simulink model "Bands2"  (R2018a)
settings: Solver=VariableStepAuto  StartTime=0.0  StopTime=0.001  RelTol=1e-3
undefined symbols (not defined in the file): fdesignblkfcn, G1, G2, gcbh, get, T
libraries: dspsrcs4 x1, dspxfrm3 x1, dspobslib x1
settings Model: Creator=Daniel  LastModifiedBy=Daniel

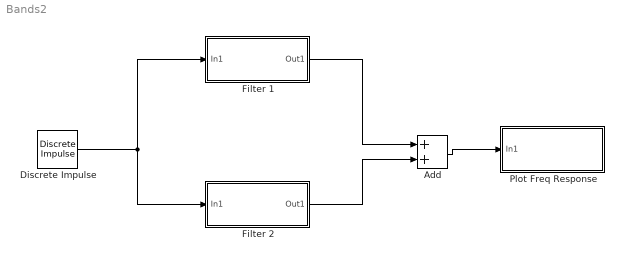
== system Bands2 ==
  Add : Sum
  Discrete Impulse : dspsrcs4/Discrete  Impulse  Delay=0  SampleTime=T  FrameSample=128  OutputFrames=off  dataType=double  isSigned=on  wordLen=16  udDataType=sfix(16)  fracBitsMode=Best precision  numFracBits=15  OutDataTypeStr=double  LastOutDataTypeStr=double
  Filter 1 : Subsystem
  Filter 2 : Subsystem
  Plot Freq Response : Subsystem
  wires:
  Discrete Impulse/1 -> Filter 2/1(In1), Filter 1/1(In1)
  Add/1 -> Plot Freq Response/1(In1)
  Filter 1/1(Out1) -> Add/1
  Filter 2/1(Out1) -> Add/2

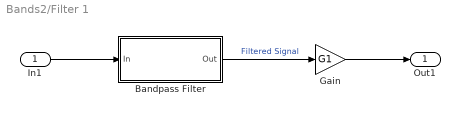
== system Bands2/Filter 1 ==
  In1 : Inport
  Bandpass Filter : Subsystem  DialogController=fdesignblkfcn  InitFcn=fdesignblkfcn(gcbh, {'InitFcn'});  mask(Bandpass Filter){}
      mask help: Design a bandpass filter
      settings: CopyFcn=fdesignblkfcn(gcbh, {'CopyFcn'});
      mask Help: helpview(mapfilelocation('dsp'), 'dspbandpassfilter');
      mask Display: disp('Bandpass');
  Gain : Gain  Gain=G1
  Out1 : Outport
  wires:
  Bandpass Filter/1(Out) -> Gain/1  "Filtered Signal"
  In1/1 -> Bandpass Filter/1(In)
  Gain/1 -> Out1/1

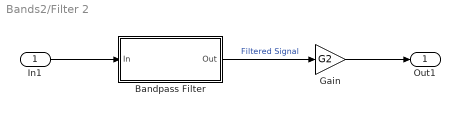
== system Bands2/Filter 2 ==
  In1 : Inport
  Bandpass Filter : Subsystem  DialogController=fdesignblkfcn  InitFcn=fdesignblkfcn(gcbh, {'InitFcn'});  mask(Bandpass Filter){}
      mask help: Design a bandpass filter
      settings: CopyFcn=fdesignblkfcn(gcbh, {'CopyFcn'});
      mask Help: helpview(mapfilelocation('dsp'), 'dspbandpassfilter');
      mask Display: disp('Bandpass');
  Gain : Gain  Gain=G2
  Out1 : Outport
  wires:
  Bandpass Filter/1(Out) -> Gain/1  "Filtered Signal"
  In1/1 -> Bandpass Filter/1(In)
  Gain/1 -> Out1/1

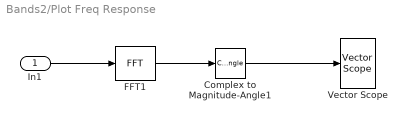
== system Bands2/Plot Freq Response ==
  In1 : Inport
  Complex to Magnitude-Angle1 : ComplexToMagnitudeAngle  Output=Magnitude
  FFT1 : dspxfrm3/FFT  FFTImplementation=Auto  CompMethod=Table lookup  TableOpt=NEW  TableOptActive=Speed  BitRevOrder=off  Normalize=off  InheritFFTLength=on  FFTLength=64  WrapInput=on  roundingMode=Floor  overflowMode=off  firstCoeffDataTypeStr=Inherit: Same word length as input  firstCoeffLastDataTypeStr=Inherit: Same word length as input  outputMin=[]  outputMax=[]
  Vector Scope : dspobslib/Vector Scope  ScopeProperties=off  Domain=Frequency  HorizSpan=1  DisplayProperties=off  AxisGrid=on  Memory=off  FrameNumber=off  AxisLegend=off  AxisZoom=off  OpenScopeAtSimStart=on  OpenScopeImmediately=off  FigPos=get(0,'defaultfigureposition')  AxisProperties=on  XUnits=Hertz  XRange=[0...Fs/2]  InheritXIncr=on  XIncr=1  XLabel=Samples  XLimit=Auto  XMin=0  XMax=1  XStart=0  YUnits=dB  YLabel=|Magnitude (dB)|  LineProperties=off  XAxisParamsVer=6.9
      settings: SourceProductName=DSP System Toolbox  SourceProductBaseCode=DS  YMin=0.0723692553519949  YMax=69.3188381671759
  wires:
  In1/1 -> FFT1/1
  FFT1/1 -> Complex to Magnitude-Angle1/1
  Complex to Magnitude-Angle1/1 -> Vector Scope/1

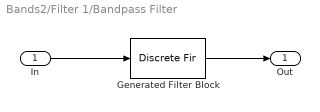
== system Bands2/Filter 1/Bandpass Filter ==
  In : Inport
  Generated Filter Block : DiscreteFir  Tag=BlockMethodSubSystem  Coefficients=[0.00263153159801553802 -0.000925904745237847958 -0.000752953473169977374 0.00300964181423011038 0.00946193180662700632 0.013265239771152652 0.0101016095527189133 0.00224346218802161683 -0.00313551560182016853 -0.00182553027462669759 0.00278714946480265735 0.00425556872385676223 0.00115409424020770121 -0.0016826234776469765 -0.000143014286550564862 0.00343941682014496392 0.0037412759983621478 9.13237388442903614e-05 -0.00245890642633806496 -0.00030933923546227495 0.00338057529801455816 0.00303982786606829926 -0.00127169553996156568 -0.00367097037971243463 -0.000795800286650436613 0.00311830911535596056 0.00203775820362573409 -0.00309021359597200619 -0.00530875958313432091 -0.00153884025574830326 0.0026371080384279765 0.000662253297386015786 -0.00538772777432254546 -0.00729726977559988586 -0.00243878935490489564 0.00197813593653708639 -0.00111562853098350588 -0.00819063882110392105 -0.00960235129002771567 -0.00341229973325703814 0.00120413112710167748 -0.00326750092556750806 -0.0114479445703728963 -0.0120834184713225126 -0.00427126300065466639 0.000436601366682421409 -0.00579826992728139576 -0.0151943158290235025 -0.0146723874270309369 -0.0048337749384548441 -0.0001706943839046445 -0.00868121376230318251 -0.0194416915082832424 -0.0172326929938897352 -0.00480858126186381289 -0.000401000231763899619 -0.0119630615008990554 -0.0243323725116025708 -0.0196319886402626098 -0.00372371315363906547 0.000106708425843307295 -0.0158134346593733176 -0.0302821814213769004 -0.0217405632821891931 -0.000703743489364856527 0.0020149354341453601 -0.0208169215753832085 -0.0385292406543400884 -0.0234407503176408821 0.00645258759694269154 0.00706733402851424369 -0.0289971431316349386 -0.0535057422705280811 -0.0246294555373343833 0.0263783898601966244 0.0229665001967281276 -0.0518982521784157949 -0.105695121198578185 -0.0252426036424847275 0.181844517790308913 0.363285121402335209 0.363285121402335209 0.181844517790308913 -0.0252426036424847275 -0.105695121198578185 -0.0518982521784157949 0.0229665001967281276 0.0263783898601966244 -0.0246294555373343833 -0.0535057422705280811 -0.0289971431316349386 0.00706733402851424369 0.00645258759694269154 -0.0234407503176408821 -0.0385292406543400884 -0.0208169215753832085 0.0020149354341453601 -0.000703743489364856527 -0.0217405632821891931 -0.0302821814213769004 -0.0158134346593733176 0.000106708425843307295 -0.00372371315363906547 -0.0196319886402626098 -0.0243323725116025708 -0.0119630615008990554 -0.000401000231763899619 -0.00480858126186381289 -0.0172326929938897352 -0.0194416915082832424 -0.00868121376230318251 -0.0001706943839046445 -0.0048337749384548441 -0.0146723874270309369 -0.0151943158290235025 -0.00579826992728139576 0.000436601366682421409 -0.00427126300065466639 -0.0120834184713225126 -0.0114479445703728963 -0.00326750092556750806 0.00120413112710167748 -0.00341229973325703814 -0.00960235129002771567 -0.00819063882110392105 -0.00111562853098350588 0.00197813593653708639 -0.00243878935490489564 -0.00729726977559988586 -0.00538772777432254546 0.000662253297386015786 0.0026371080384279765 -0.00153884025574830326 -0.00530875958313432091 -0.00309021359597200619 0.00203775820362573409 0.00311830911535596056 -0.000795800286650436613 -0.00367097037971243463 -0.00127169553996156568 0.00303982786606829926 0.00338057529801455816 -0.00030933923546227495 -0.00245890642633806496 9.13237388442903614e-05 0.0037412759983621478 0.00343941682014496392 -0.000143014286550564862 -0.0016826234776469765 0.00115409424020770121 0.00425556872385676223 0.00278714946480265735 -0.00182553027462669759 -0.00313551560182016853 0.00224346218802161683 0.0101016095527189133 0.013265239771152652 0.00946193180662700632 0.00300964181423011038 -0.000752953473169977374 -0.000925904745237847958 0.00263153159801553802]  InputProcessing=Columns as channels (frame based)
  Out : Outport
  wires:
  In/1 -> Generated Filter Block/1
  Generated Filter Block/1 -> Out/1

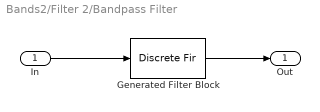
== system Bands2/Filter 2/Bandpass Filter ==
  In : Inport
  Generated Filter Block : DiscreteFir  Tag=BlockMethodSubSystem  Coefficients=[-0.00277583134256976886 0.01479724496396124 -0.0122372115988817719 -0.00179948060774227925 0.00467653679756307658 0.00553023427845650631 -0.00588174934326072749 -0.000979437037093786045 -0.00106255053392637078 0.00240347552664520181 0.0043241814452752228 -0.00467116539590085519 -0.000321320529674491706 -0.00189650625160915978 0.00225558032553131727 0.00455563441113918804 -0.00426383384311687652 -0.000255070291463620202 -0.00286459728789077023 0.00253614926023660453 0.00504376815779768867 -0.00408241250415413912 -0.000198393279908001124 -0.00409365823511384508 0.00303044167708087578 0.00559153975051013274 -0.0038887776469767911 -7.74730218718738817e-05 -0.00565124906786004105 0.0036983764677051903 0.00612573694771929161 -0.00355155690691512371 0.000130370788366439283 -0.00760546459120371374 0.00453802888577428329 0.00658304278529808426 -0.00293858894668411891 0.000404893820113830932 -0.0100077557095643727 0.0055486342101122299 0.00690212470614823964 -0.00190829468253043977 0.000723767199091361613 -0.0129400868285139796 0.00674612221442017108 0.00701596348356677869 -0.000279963555115048807 0.00106465748362582352 -0.0165361794438585105 0.008150812619645037 0.00685431267228603369 0.00220788272485532983 0.00140812601824610861 -0.0210497540774029698 0.00982064144358713899 0.0062972436272553476 0.0060172989734582176 0.00172388778676163014 -0.0269894779007830155 0.0118748939052019109 0.00515636817862194508 0.0120370492686849434 0.00201032062561973257 -0.0355621257996417139 0.0146359385154571746 0.0030026615242447945 0.0224690418873391279 0.00225298044071896297 -0.0501198145354184582 0.0190875950963904431 -0.00148346582105329805 0.044700323919381009 0.00240197374568666688 -0.0844552561293984289 0.0299323133249636622 -0.0154554596376694237 0.128107937362240437 0.00250556520919734127 -0.337126519607747421 0.240916994329211431 0.240916994329211431 -0.337126519607747421 0.00250556520919734127 0.128107937362240437 -0.0154554596376694237 0.0299323133249636622 -0.0844552561293984289 0.00240197374568666688 0.044700323919381009 -0.00148346582105329805 0.0190875950963904431 -0.0501198145354184582 0.00225298044071896297 0.0224690418873391279 0.0030026615242447945 0.0146359385154571746 -0.0355621257996417139 0.00201032062561973257 0.0120370492686849434 0.00515636817862194508 0.0118748939052019109 -0.0269894779007830155 0.00172388778676163014 0.0060172989734582176 0.0062972436272553476 0.00982064144358713899 -0.0210497540774029698 0.00140812601824610861 0.00220788272485532983 0.00685431267228603369 0.008150812619645037 -0.0165361794438585105 0.00106465748362582352 -0.000279963555115048807 0.00701596348356677869 0.00674612221442017108 -0.0129400868285139796 0.000723767199091361613 -0.00190829468253043977 0.00690212470614823964 0.0055486342101122299 -0.0100077557095643727 0.000404893820113830932 -0.00293858894668411891 0.00658304278529808426 0.00453802888577428329 -0.00760546459120371374 0.000130370788366439283 -0.00355155690691512371 0.00612573694771929161 0.0036983764677051903 -0.00565124906786004105 -7.74730218718738817e-05 -0.0038887776469767911 0.00559153975051013274 0.00303044167708087578 -0.00409365823511384508 -0.000198393279908001124 -0.00408241250415413912 0.00504376815779768867 0.00253614926023660453 -0.00286459728789077023 -0.000255070291463620202 -0.00426383384311687652 0.00455563441113918804 0.00225558032553131727 -0.00189650625160915978 -0.000321320529674491706 -0.00467116539590085519 0.0043241814452752228 0.00240347552664520181 -0.00106255053392637078 -0.000979437037093786045 -0.00588174934326072749 0.00553023427845650631 0.00467653679756307658 -0.00179948060774227925 -0.0122372115988817719 0.01479724496396124 -0.00277583134256976886]  InputProcessing=Columns as channels (frame based)
  Out : Outport
  wires:
  In/1 -> Generated Filter Block/1
  Generated Filter Block/1 -> Out/1
